simulink model "smib_optimized"  (R2015b)
settings: Solver=ode45  SolverMode=SingleTasking  StartTime=0.0  StopTime=30  RelTol=1e-4
undefined symbols (not defined in the file or in its folder): D1, Delta
libraries: powerlib x12, powerlib_meascontrol x1, sps_avr x1
settings Model: Creator=user  LastModifiedBy=mluser
settings DataIOCC: LimitDataPoints=off
settings DebuggingCC: AllowSymbolicDim=on  SFUnexpectedBacktrackingDiag=error  SFNoUnconditionalDefaultTransitionDiag=error
settings ModelReferenceCC: PropagateSignalLabelsOutOfModel=on
settings SFSimCC: SimUseLocalCustomCode=on
settings RTWCC: RTWUseLocalCustomCode=on
settings GRTTargetCC: TargetLangStandard=C99 (ISO)
settings ConfigComp: CovMetricSettings=dwe  CovSaveCumulativeToWorkspaceVar=off  CovSaveSingleToWorkspaceVar=off  CovModelRefEnable=Off  CovExternalEMLEnable=on

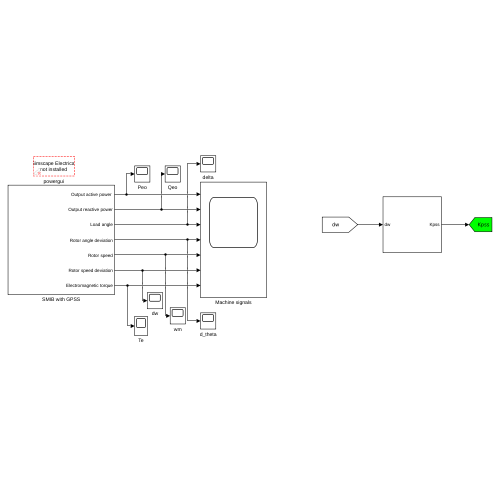
[thumbnail: Simulink's stored preview of the top-level diagram]
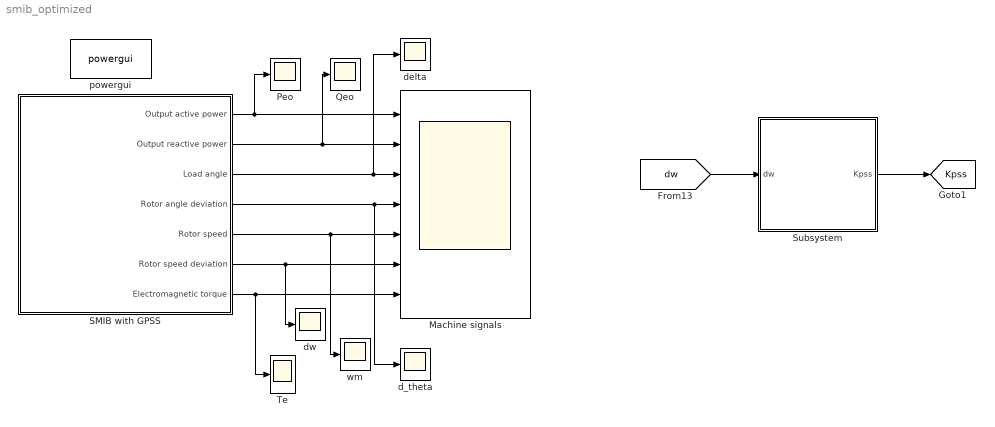
== system smib_optimized ==
  Machine signals : Scope  NumInputPorts=7
  Peo : Scope
  Qeo : Scope
  SMIB with GPSS : Subsystem
  Subsystem : Subsystem
  Te : Scope
  d_theta : Scope
  delta : Scope
  dw : Scope
  powergui : powerlib/powergui  Priority=1  SimulationMode=Phasor  SampleTime=50e-6  frequency=60  Iterations=50  frequencyindice=60  Pbase=100e6  ErrMax=0.0001  UnitsV=kV  UnitsW=MW  buscounter=0  FunctionMessages=off  echomessages=off  EnableUseOfTLC=off  CurrentSourceSwitches=off  DisableSnubberDevices=off  DisableRonSwitches=off  DisableVfSwitches=off  DisplayEquations=off  SolverType=Tustin/Backward Euler (TBE)  Interpol=off  ExternalGateDelay=off  methode=off  Ts=100  x0status=blocks  SPID=on  SwTol=0  HookPort=off  RestoreLinks=warning  ResistiveCurrentMeasurement=off  Frange=[0:2:500]  Ylog=off  Xlog=on  ShowGrid=off  save=off  variable=ZData  structure=0  ZoomFFT=off  StartTime=0.0  cycles=1  DisplayStyle=1  fundamental=60  FreqAxis=off  MaxFrequency=1000  frequencyindicesteady=1  RmsSteady=1  display=off
  wm : Scope
  tag scope: Kpss=global
  wires:
  SMIB with GPSS/5(Rotor speed) -> wm/1, Machine signals/5
  SMIB with GPSS/1("Output active power ") -> Peo/1, Machine signals/1
  SMIB with GPSS/4(Rotor angle deviation) -> d_theta/1, Machine signals/4
  SMIB with GPSS/3(Load angle) -> delta/1, Machine signals/3
  SMIB with GPSS/7(Electromagnetic torque) -> Machine signals/7, Te/1
  SMIB with GPSS/2(Output reactive power) -> Qeo/1, Machine signals/2
  SMIB with GPSS/6(Rotor speed deviation) -> dw/1, Machine signals/6
  [dw] -> Subsystem/1(dw)
  Subsystem/1(Kpss) -> [Kpss]

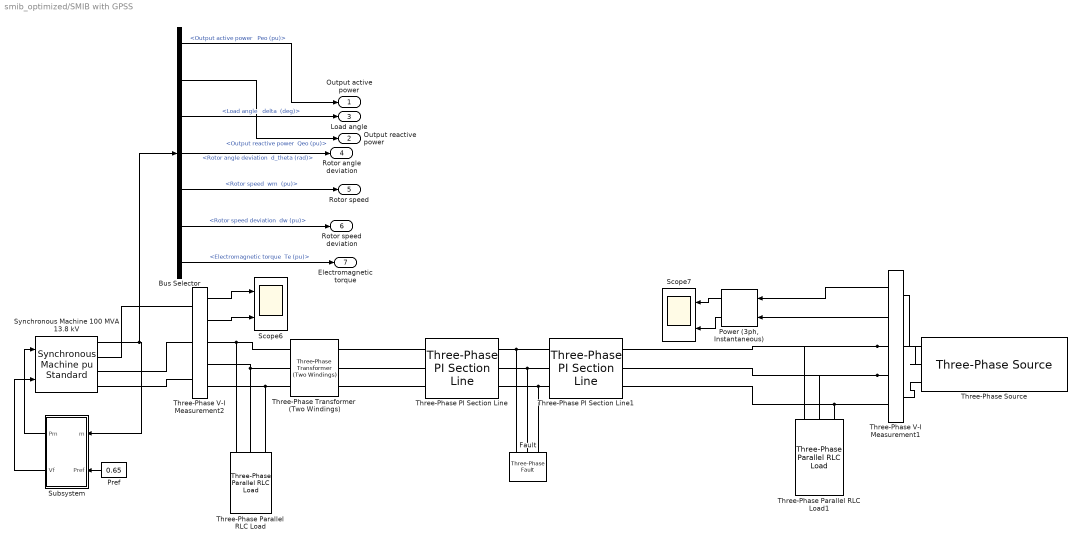
== system smib_optimized/SMIB with GPSS ==
  Bus Selector : BusSelector  OutputSignals="Output active power   Peo (pu),Output reactive power  Qeo (pu),Load angle   delta  (deg),Mechanical.Rotor angle deviation  d_theta (rad),Mechanical.Rotor speed  wm  (pu),Mechanical.Rotor speed deviation  dw (pu),Mechanical.Electromagnetic torque  Te (pu)"
  Fault : powerlib/Elements/Three-Phase Fault  InitialStates=0  FaultA=on  FaultB=on  FaultC=on  GroundFault=on  SwitchTimes=[ 3 3+12/60]  External=off  SwitchStatus=NaN  FaultResistance=0.001  GroundResistance=0.001  SnubberResistance=inf  SnubberCapacitance=0  Measurements=None
  "Power (3ph, Instantaneous)" : powerlib_meascontrol/Measurements/Power (3ph, Instantaneous)
  Pref : Constant  Value=0.65
  Scope6 : Scope  NumInputPorts=2
  Scope7 : Scope  NumInputPorts=2
  Subsystem : Subsystem
  Synchronous Machine 100 MVA 13.8 kV : powerlib/Machines/Synchronous Machine pu Standard  PresetModel=No  MechanicalLoad=Mechanical power Pm  ShowDetailedParameters=on  RotorType=Salient-pole  Units=per unit standard parameters  MeasurementBus=off  NominalParameters="[ 100E6  13800   60 ]"  Reactances1=[ 31 32 33 34 35 36 37 ]  Reactances2=[ 1.305, 0.296, 0.252, 0.474, 0.243, 0.18 ]  dAxisTimeConstants=Short-circuit  qAxisTimeConstants=Open-circuit  TimeConstants1=[]  TimeConstants2=[]  TimeConstants3=[]  TimeConstants4=[]  TimeConstants5=[ 1.01, 0.053, 0.1 ]  TimeConstants6=[]  TimeConstants7=[]  TimeConstants8=[]  StatorResistance=2.8544e-3  Mechanical=[ 3.2 0 2]  PolePairs=2  InitialConditions=[0 -51.4809 0.623758 0.623758 0.623758 11.3333 -108.667 131.333 1.41031]  SetSaturation=off  Saturation=[0.6404,0.7127,0.8441,0.9214,0.9956,1.082,1.19,1.316,1.457;0.7,0.7698,0.8872,0.9466,0.9969,1.046,1.1,1.151,1.201]  LoadFlowParameters=[4 65000000 0 0 15000000]  TsPowergui=0  TsBlock=-1  IterativeModel=Trapezoidal non iterative  IterativeDiscreteModel=Trapezoidal non iterative  BusType=PQ  Pref=65e6  Qref=15e6  Qmin=-Inf  Qmax=Inf  PLF=0  QLF=0
      settings: AttributesFormatString=\n\n
  Three-Phase PI Section Line : powerlib/Elements/Three-Phase PI Section Line  LConnTagsString=a|b|c  RConnTagsString=A|B|C  Frequency=60  Resistances=[ 0.225 0.675]  Inductances="[ 1.7913e-3  5.373e-3]"  Capacitances=[6.4e-9 19.2e-9]  Length=47
  Three-Phase PI Section Line1 : powerlib/Elements/Three-Phase PI Section Line  LConnTagsString=a|b|c  RConnTagsString=A|B|C  Frequency=60  Resistances=[ 0.225 0.675]  Inductances="[ 1.7913e-3  5.373e-3]"  Capacitances=[6.4e-9 19.2e-9]  Length=47
  Three-Phase Parallel RLC Load : powerlib/Elements/Three-Phase Parallel RLC Load  LConnTagsString=A|B|C  Configuration=Y (grounded)  NominalVoltage=13800  Vabc=[1e3 1e3 1e3]  Vabcp=[1e3 1e3 1e3]  NominalFrequency=60  UnbalancedPower=off  ActivePower=40e6  InductivePower=15e6  CapacitivePower=0  Pabc=[10e3 9e3 11e3]  QLabc=[100 90 110]  QCabc=[100 90 110]  Pabcp=[10e3 9e3 11e3]  QLabcp=[100 90 110]  QCabcp=[100 90 110]  Measurements=None  LoadType=constant Z
  Three-Phase Parallel RLC Load1 : powerlib/Elements/Three-Phase Parallel RLC Load  LConnTagsString=A|B|C  Configuration=Y (grounded)  NominalVoltage=230e3  Vabc=[1e3 1e3 1e3]  Vabcp=[1e3 1e3 1e3]  NominalFrequency=60  UnbalancedPower=off  ActivePower=25e6  InductivePower=0  CapacitivePower=0  Pabc=[10e3 9e3 11e3]  QLabc=[100 90 110]  QCabc=[100 90 110]  Pabcp=[10e3 9e3 11e3]  QLabcp=[100 90 110]  QCabcp=[100 90 110]  Measurements=None  LoadType=constant Z
  Three-Phase Transformer (Two Windings) : powerlib/Elements/Three-Phase Transformer (Two Windings)  Winding1Connection=Yg  Winding2Connection=Delta (D1)  CoreType=Three single-phase transformers  SetSaturation=off  Hysteresis=off  DataFile='hysteresis'  SetInitialFlux=off  Measurements=None  UNITS=pu  NominalPower=[ 1000e6 , 60 ]  Winding1=[ 13800 , 0.002 , 0.08 ]  Winding2=[ 230e3 , 0.002 , 0.08 ]  Rm=500  Lm=500  L0=0.5  Saturation=[ 0,0 ; 0.0024,1.2 ; 1.0,1.52 ]  InitialFluxes=[ 0.8 , -0.8 , 0.7 ]  MoreParameters=off  BreakLoop=off  DataType=off  TransfoNumber=1
  Three-Phase V-I Measurement1 : powerlib/Measurements/Three-Phase V-I Measurement  VoltageMeasurement=phase-to-ground  SetLabelV=off  LabelV=Vabc  Vpu=off  VpuLL=off  CurrentMeasurement=yes  SetLabelI=off  LabelI=Iabc  Ipu=off  Pbase=100e6  Vbase=500e3  OutputType=Complex  PhasorSimulation=on  PSBequivalent=0
  Three-Phase V-I Measurement2 : powerlib/Measurements/Three-Phase V-I Measurement  VoltageMeasurement=phase-to-ground  SetLabelV=off  LabelV=Vabc  Vpu=off  VpuLL=off  CurrentMeasurement=yes  SetLabelI=off  LabelI=Iabc  Ipu=off  Pbase=100e6  Vbase=500e3  OutputType=Complex  PhasorSimulation=on  PSBequivalent=0
  Three-Phase Source : powerlib/Electrical Sources/Three-Phase Source  InternalConnection=Yg  VoltagePhases=off  Voltage=230e3  PhaseAngle=0  Voltage_phases=[25e3 25e3 25e3]/sqrt(3)  PhaseAngles_phases=[0 -120 +120]  Frequency=60  NonIdealSource=on  SpecifyImpedance=on  Resistance=0.8929  Inductance=16.58e-3  ShortCircuitLevel=100e6  BaseVoltage=230e3  XRratio=7  BusType=swing  Pref=10e3  Qref=0  Prefabc=[10e3, 10e3, 10e3]  Qrefabc=[0, 0, 0]  Qmin=-inf  Qmax=inf
  "Output active power " : Outport
  Output reactive power : Outport  Port=2
  Load angle : Outport  Port=3
  Rotor angle deviation : Outport  Port=4
  Rotor speed : Outport  Port=5
  Rotor speed deviation : Outport  Port=6
  Electromagnetic torque : Outport  Port=7
  wires:
  Synchronous Machine 100 MVA 13.8 kV/1 -> Bus Selector/1, Subsystem/1(m)
  Subsystem/1(Pm) -> Synchronous Machine 100 MVA 13.8 kV/1
  Subsystem/2(Vf) -> Synchronous Machine 100 MVA 13.8 kV/2
  Pref/1 -> Subsystem/2(Pref)
  Bus Selector/1 -> "Output active power "/1  "<Output active power   Peo (pu)>"
  Bus Selector/2 -> Output reactive power/1  "<Output reactive power  Qeo (pu)>"
  Bus Selector/3 -> Load angle/1  "<Load angle   delta  (deg)>"
  Bus Selector/4 -> Rotor angle deviation/1  "<Rotor angle deviation  d_theta (rad)>"
  Bus Selector/5 -> Rotor speed/1  "<Rotor speed  wm  (pu)>"
  Bus Selector/6 -> Rotor speed deviation/1  "<Rotor speed deviation  dw (pu)>"
  Bus Selector/7 -> Electromagnetic torque/1  "<Electromagnetic torque  Te (pu)>"
  Three-Phase V-I Measurement2/2 -> Scope6/2
  Three-Phase V-I Measurement2/1 -> Scope6/1
  "Power (3ph, Instantaneous)"/2 -> Scope7/2
  Three-Phase V-I Measurement1/2 -> "Power (3ph, Instantaneous)"/2
  Three-Phase V-I Measurement1/1 -> "Power (3ph, Instantaneous)"/1
  "Power (3ph, Instantaneous)"/1 -> Scope7/1
  connections:
  Three-Phase Transformer (Two Windings)/LConn2 -- Three-Phase Parallel RLC Load/LConn2 -- Three-Phase V-I Measurement2/RConn2
  Three-Phase Parallel RLC Load/LConn1 -- Three-Phase Transformer (Two Windings)/LConn1 -- Three-Phase V-I Measurement2/RConn1
  Three-Phase V-I Measurement2/RConn3 -- Three-Phase Parallel RLC Load/LConn3 -- Three-Phase Transformer (Two Windings)/LConn3
  Three-Phase PI Section Line/LConn1 -- Three-Phase Transformer (Two Windings)/RConn1
  Three-Phase PI Section Line/LConn3 -- Three-Phase Transformer (Two Windings)/RConn3
  Three-Phase PI Section Line/LConn2 -- Three-Phase Transformer (Two Windings)/RConn2
  Synchronous Machine 100 MVA 13.8 kV/RConn1 -- Three-Phase V-I Measurement2/LConn1
  Synchronous Machine 100 MVA 13.8 kV/RConn2 -- Three-Phase V-I Measurement2/LConn2
  Synchronous Machine 100 MVA 13.8 kV/RConn3 -- Three-Phase V-I Measurement2/LConn3
  Three-Phase PI Section Line1/LConn1 -- Three-Phase PI Section Line/RConn1 -- Fault/LConn1
  Three-Phase PI Section Line1/LConn3 -- Three-Phase PI Section Line/RConn3 -- Fault/LConn3
  Three-Phase V-I Measurement1/RConn1 -- Three-Phase PI Section Line1/RConn1 -- Three-Phase Parallel RLC Load1/LConn1
  Three-Phase PI Section Line1/RConn3 -- Three-Phase Parallel RLC Load1/LConn3 -- Three-Phase V-I Measurement1/RConn3
  Three-Phase PI Section Line1/LConn2 -- Fault/LConn2 -- Three-Phase PI Section Line/RConn2
  Three-Phase V-I Measurement1/RConn2 -- Three-Phase PI Section Line1/RConn2 -- Three-Phase Parallel RLC Load1/LConn2
  Three-Phase Source/RConn1 -- Three-Phase V-I Measurement1/LConn1
  Three-Phase Source/RConn2 -- Three-Phase V-I Measurement1/LConn2
  Three-Phase Source/RConn3 -- Three-Phase V-I Measurement1/LConn3

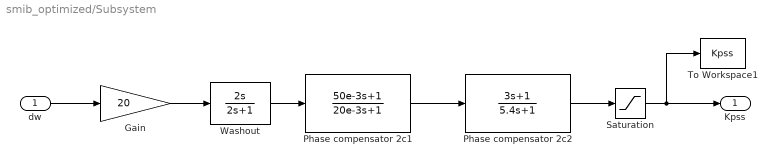
== system smib_optimized/Subsystem ==
  dw : Inport
  Gain : Gain  Gain=20
  "Phase compensator 2c1 " : TransferFcn  Numerator=[50e-3 1]  Denominator=[20e-3 1]
  Phase compensator 2c2 : TransferFcn  Numerator=[3 1]  Denominator=[5.4 1]
  Saturation : Saturate
  To Workspace1 : ToWorkspace  VariableName=Kpss  SampleTime=-1
  "Washout " : TransferFcn  Numerator=[2 0]  Denominator=[2 1]
  Kpss : Outport
  wires:
  Gain/1 -> "Washout "/1
  dw/1 -> Gain/1
  Saturation/1 -> Kpss/1, To Workspace1/1
  "Washout "/1 -> "Phase compensator 2c1 "/1
  "Phase compensator 2c1 "/1 -> Phase compensator 2c2/1
  Phase compensator 2c2/1 -> Saturation/1

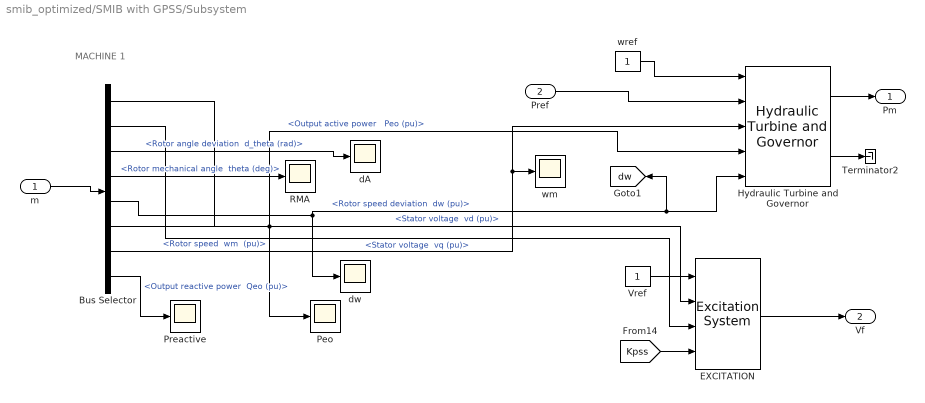
== system smib_optimized/SMIB with GPSS/Subsystem ==
  note: MACHINE 1
  m : Inport
  Pref : Inport  Port=2
  Bus Selector : BusSelector  OutputSignals="dq0 components.Stator voltage  vd (pu),dq0 components.Stator voltage  vq (pu),Mechanical.Rotor angle deviation  d_theta (rad),Mechanical.Rotor mechanical angle  theta (deg),Mechanical.Rotor speed deviation  dw (pu),Output active power   Peo (pu),Mechanical.Rotor speed  wm  (pu),Output reactive power  Qeo (pu)"
  EXCITATION : sps_avr/Excitation System  tr=20e-3  reg=[ 400, 0.025 ]  exc=[ 1, 0 ]  tgr=[ 0, 0 ]  damp=[ 0, 0 ]  sat=[ 0, 0 ]  lim=[ 0 , 12.3, 0 ]  v0=[1,1.41031]
  Hydraulic Turbine and Governor : powerlib/Machines/Hydraulic Turbine and Governor  sm="[ 10/3  0.07 ]"  gate="[  0.01  0.97518  -0.1  0.1 ]"  reg="[  0.05  1.163  0.105  0  0.01  ]"  hyd="[  0  2.67  ]"  dref=0  po=0.651111
  Peo : Scope
  Preactive : Scope
  RMA : Scope
  Terminator2 : Terminator
  Vref : Constant
  dA : Scope
  dw : Scope
  wm : Scope
  wref : Constant
  Pm : Outport  InitialOutput=0
  Vf : Outport  Port=2  InitialOutput=0
  tag scope: dw=global
  wires:
  EXCITATION/1 -> Vf/1
  wref/1 -> Hydraulic Turbine and Governor/1
  Bus Selector/3 -> dA/1  "<Rotor angle deviation  d_theta (rad)>"
  Bus Selector/1 -> EXCITATION/2  "<Stator voltage  vd (pu)>"
  m/1 -> Bus Selector/1
  Bus Selector/2 -> EXCITATION/3  "<Stator voltage  vq (pu)>"
  Pref/1 -> Hydraulic Turbine and Governor/2
  Vref/1 -> EXCITATION/1
  Bus Selector/4 -> RMA/1  "<Rotor mechanical angle  theta (deg)>"
  Hydraulic Turbine and Governor/1 -> Pm/1
  Hydraulic Turbine and Governor/2 -> Terminator2/1
  Bus Selector/5 -> dw/1, [dw], Hydraulic Turbine and Governor/5  "<Rotor speed deviation  dw (pu)>"
  Bus Selector/6 -> Peo/1, Hydraulic Turbine and Governor/4  "<Output active power   Peo (pu)>"
  Bus Selector/7 -> Hydraulic Turbine and Governor/3, wm/1  "<Rotor speed  wm  (pu)>"
  Bus Selector/8 -> Preactive/1  "<Output reactive power  Qeo (pu)>"
  [Kpss] -> EXCITATION/4
